simulink model "part1q3"  (R2023a)
settings: Solver=VariableStepAuto  StartTime=0.0  StopTime=0.1  RelTol=1e-3
libraries: dspfdesign x1
settings Model: Creator=J_MEHMAN  LastModifiedBy=J_MEHMAN

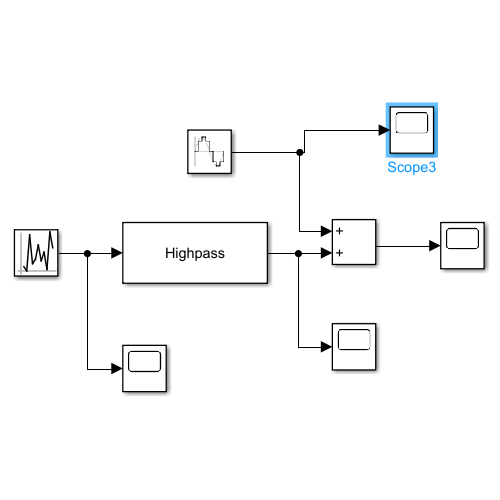
[thumbnail: Simulink's stored preview of the top-level diagram]
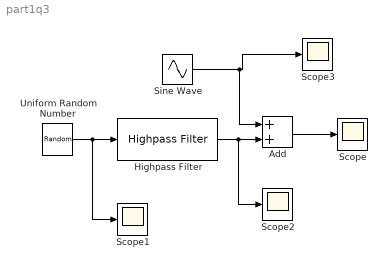
== system part1q3 ==
  Add : Sum
  Highpass Filter : dspfdesign/Highpass Filter  FilterType=IIR  DesignForMinimumOrder=on  FilterOrder=50  StopbandFrequency=3600  PassbandFrequency=3800  StopbandAttenuation=60  PassbandRipple=1  SampleRateMode=Specify on dialog  SampleRate=8000  SimulateUsing=Interpreted execution  roundingMode=Floor  coeffsDataTypeStr=fixdt(1,16)
  Scope{,1..3} (4 alike) : Scope
  Sine Wave : Sin  Frequency=100*2*pi  Samples=100  SampleTime=1/8000
  Uniform Random Number : UniformRandomNumber  Minimum=-5  Maximum=5  SampleTime=1/8000
  wires:
  Sine Wave/1 -> Scope3/1, Add/1
  Highpass Filter/1 -> Scope2/1, Add/2
  Add/1 -> Scope/1
  Uniform Random Number/1 -> Scope1/1, Highpass Filter/1
